simulink model "Measure_BH_curve2"  (R2016a)
settings: Solver=ode23tb  StartTime=0.0  StopTime=1  RelTol=1e-3
libraries: powerlib x9, simulink x1
settings Model: Creator=Administrator  LastModifiedBy=Administrator
settings DataIOCC: LimitDataPoints=on  SaveFormat=Array
settings DebuggingCC: SolverPrmCheckMsg=warning
settings HardwareCC: ProdBitPerPointer=32  ProdLargestAtomicFloat=None  ProdIntDivRoundTo=Undefined  ProdEndianess=Unspecified  ProdWordSize=32  ProdHWDeviceType=32-bit Generic
settings ModelReferenceCC: PropagateSignalLabelsOutOfModel=off
settings ConfigComp: CovModelRefEnable=Off  CovSFcnEnable=off

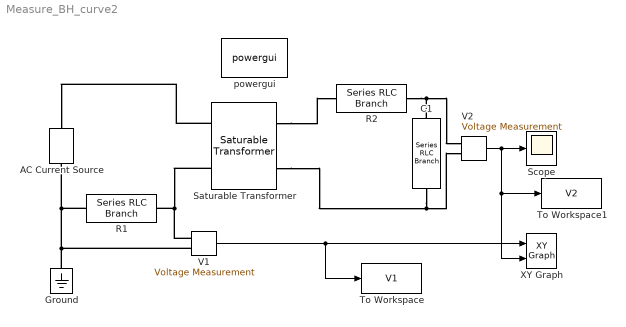
== system Measure_BH_curve2 ==
  AC Current Source : powerlib/Electrical Sources/AC Current Source  Amplitude=10  Phase=90  Frequency=50  SampleTime=0  Measurements=None
  C1 : powerlib/Elements/Series RLC Branch  LConnTagsString=__new0  RConnTagsString=__new0  BranchType=C  Resistance=1  Inductance=1e-3  SetiL0=off  InitialCurrent=0  Capacitance=10e-6  Setx0=off  InitialVoltage=430  Measurements=None
  Ground : powerlib/Elements/Ground  LConnTagsString=a
  R1 : powerlib/Elements/Series RLC Branch  LConnTagsString=__new0  RConnTagsString=__new0  BranchType=R  Resistance=1  Inductance=1e-3  SetiL0=off  InitialCurrent=0  Capacitance=1e-6  Setx0=off  InitialVoltage=0  Measurements=None
  R2 : powerlib/Elements/Series RLC Branch  LConnTagsString=__new0  RConnTagsString=__new0  BranchType=R  Resistance=400e3  Inductance=1e-3  SetiL0=off  InitialCurrent=0  Capacitance=1e-6  Setx0=off  InitialVoltage=0  Measurements=None
  Saturable Transformer : powerlib/Elements/Saturable Transformer  ThreeWindings=off  Hysteresis=on  DataFile='my_hysteresis.mat'  Measurements=None  UNITS=pu  NominalPower=[250e6 50]  Winding1="[ 735e3  0.002  0 ]"  Winding2="[ 315e3  0.002  0.08 ]"  Winding3="[ 315e3  0.002  0.08 ]"  Saturation=[ 0,0 ; 0.0024,1.2 ; 1.0,1.52 ]  CoreLoss=[500]  MoreParameters=off  BreakLoop=on  DataType=off  InitialFlux=-5.46086292085219  TransfoNumber=1
  Scope : Scope
  To Workspace : ToWorkspace  VariableName=V1  SampleTime=-1
      settings: Save2DSignal=2-D array (concatenate along first dimension)
  To Workspace1 : ToWorkspace  VariableName=V2  SampleTime=-1
      settings: Save2DSignal=2-D array (concatenate along first dimension)
  V1 : powerlib/Measurements/Voltage Measurement  PhasorSimulation=off  OutputType=Complex  PSBequivalent=0
  V2 : powerlib/Measurements/Voltage Measurement  PhasorSimulation=off  OutputType=Complex  PSBequivalent=0
  XY Graph : simulink/Sinks/XY Graph  xmin=-2e1  xmax=2e1  ymin=-6e2  ymax=6e2  st=-1
  powergui : powerlib/powergui  Priority=1  SimulationMode=Discrete  SolverType=Tustin  SampleTime=50e-6  frequency=60  SPID=off  DisableSnubberDevices=off  DisableRonSwitches=off  DisableVfSwitches=off  SwTol=0  DisplayEquations=off  Interpol=off  ExternalGateDelay=off  methode=off  Ts=0  FunctionMessages=off  echomessages=off  HookPort=off  EnableUseOfTLC=off  x0status=blocks  frequencyindice=0  Pbase=100e6  ErrMax=1e-4  Iterations=50  UnitsV=kV  UnitsW=MW  buscounter=0  RestoreLinks=warning  ResistiveCurrentMeasurement=off  Frange=[0:2:500]  Ylog=off  Xlog=on  ShowGrid=off  save=off  variable=ZData  structure=0  ZoomFFT=off  StartTime=0.0  cycles=1  DisplayStyle=1  fundamental=60  FreqAxis=off  MaxFrequency=1000  frequencyindicesteady=1  RmsSteady=1  display=off
  wires:
  V1/1 -> To Workspace/1, XY Graph/1
  V2/1 -> XY Graph/2, To Workspace1/1, Scope/1
  connections:
  Saturable Transformer/RConn2 -- C1/RConn1 -- V2/LConn2
  Ground/LConn1 -- R1/LConn1 -- AC Current Source/LConn1 -- V1/LConn2
  V1/LConn1 -- Saturable Transformer/LConn2 -- R1/RConn1
  R2/RConn1 -- C1/LConn1 -- V2/LConn1
  Saturable Transformer/LConn1 -- AC Current Source/RConn1
  Saturable Transformer/RConn1 -- R2/LConn1
